simulink model "HLS_VMC_testing"  (R2025a)
settings: Solver=VariableStepAuto  StartTime=0.0  StopTime=0.0001  RelTol=1e-3
InitFcn:
  | fs = 500e6;
values from neighbouring files (symbols this model uses):
  N = length(X)    [outputPlots.m]
undefined symbols (not defined in the file or in its folder): A, es1, i, S, vsva2488, xcvr1602
libraries: hdlBasic x98, hlsBasic x64, aieUtilities x18, dspsrcs4 x15, dspxfrm3 x2, hdlDSPIP x2, hlsUtilities x1, vmcUtilities x1
(part 3 of 4)

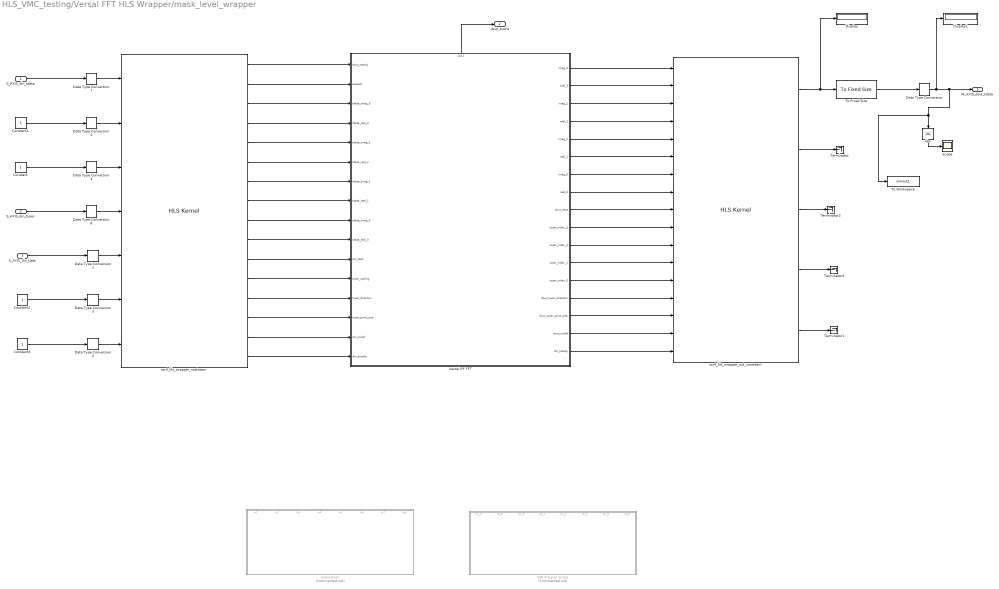
== system HLS_VMC_testing/Versal FFT HLS Wrapper/mask_level_wrapper ==
  S_AXIS_din_tdata : Inport
  S_AXIS_din_tuser : Inport  Port=2
  S_AXIS_din_tlast : Inport  Port=3
  Abs : Abs  SaturateOnIntegerOverflow=off
  Constant{,1..3} (4 alike) : Constant
  Data Type Conversion : hlsBasic/Data Type Conversion  OutDataType=double  TypeExp=''  Signedness=Signed  WordLength=16  FractionalLength=0  RoundingMode=Truncation to minus infinity  OverflowMode=Wrap around
  Data Type Conversion{1..5} (5 alike) : hlsBasic/Data Type Conversion  OutDataType=data type expression  TypeExp='x_ufix1'  Signedness=Signed  WordLength=16  FractionalLength=0  RoundingMode=Truncation to minus infinity  OverflowMode=Wrap around
  Data Type Conversion7 : hlsBasic/Data Type Conversion  OutDataType=data type expression  TypeExp='x_sfix64_En63'  Signedness=Signed  WordLength=16  FractionalLength=0  RoundingMode=Truncation to minus infinity  OverflowMode=Wrap around  SaturateOnIntegerOverflow=on
  Data Type Conversion8 : hlsBasic/Data Type Conversion  OutDataType=data type expression  TypeExp='x_ufix18'  Signedness=Signed  WordLength=16  FractionalLength=0  RoundingMode=Truncation to minus infinity  OverflowMode=Wrap around
  Display : Display
  Display1 : Display
  SSR 4 Signal Scope : Subsystem  Commented=on
  Scope : Scope
      settings: ActiveDisplayYMinimum=-0.036579755749096929  ActiveDisplayYMaximum=0.32921780174187243  DataLoggingVariableName=ScopeData4
  Subsystem : Subsystem  Commented=on
  Terminator{,1..3} (4 alike) : Terminator
  To Fixed Size : aieUtilities/To Fixed Size  Mode=Stop simulation when input variable-size signal is not full  OutputSize=Inherit: Same as input  CopyMethod=Buffer samples to form output  HasStatusOutput=on
  To Workspace : ToWorkspace  VariableName=simout1  SaveFormat=Timeseries  SampleTime=-1
  Versal RF FFT : Subsystem
      settings: PortSchema="{\"entries\":[{\"content\":{\"sides\":[{\"content\":{\"connectorIds\":[\"In1\",\"In2\",\"In3\",\"In4\",\"In5\",\"In6\",\"In7\",\"In8\",\"In9\",\"In10\",\"In11\",\"In12\",\"In13\",\"In14\",\"In15\",\"In16\"]},\"type\":\"ConnectorPlacement.EquallySpacedRectSide\",\"uuid\":\"209a2209-87d3-42b4-b17f-a75cbba28a6a\"},{\"content\":{\"connectorIds\":[\"Out1\",\"Out2\",\"Out3\",\"Out4\",\"Out5\",\"Out6\",\"Out7\",\"Out8\",\"Out9\",\"Out10\",\"Out11\",\"Out12\",\"Out13\",\"Out14\",\"Out15\",\"Out16\",\"Out17\"],\"side\":\"RIGHT\"},\"type\":\"ConnectorPlacement.EquallySpacedRectSide\",\"uuid\":\"ba4fa1b1-993b-4b6c-82ac-7a0960139a7d\"},{\"content\":{\"connectorIds\":[\"Out18\"],\"side\":\"TOP\"},\"type\":\"ConnectorPlacement.EquallySpacedRectSide\",\"uuid\":\"00677fce-2a91-4297-b798-cc966ff20102\"}]},\"type\":\"ConnectorPlacement.EquallySpacedConnector\",\"uuid\":\"b06fffb5-4716-4994-a196-524358a0c89f\"}],\"packageUris\":[\"http://schema.mathworks.com/mf0/Connector/R2020b\"],\"version\":\"1.0\"}"
  ssr4_hls_wrapper_nostream : hlsBasic/HLS Kernel  PortNames={'return'; 'S_AXIS_din_tdata'; 'S_AXIS_din_tready_IN'; 'S_AXIS_din_tvalid_IN'; 'S_AXIS_din_tuser_IN'; 'S_AXIS_din_tlast_IN'; 'S_AXI_aresetn_IN'; 'S_AXI_enable_IN'; 'M_AXIS_dout_tready_OUT'; 'M_AXI_aresetn_OUT'; 'M_AXIS_din_tdata_sample_3_imag'; 'M_AXIS_din_tdata_sample_3_real'; 'M_AXIS_din_tdata_sample_2_imag'; 'M_AXIS_din_tdata_sample_2_real'; 'M_AXIS_din_tdata_sample_1_imag'; 'M_AXIS_din_tdata_sample_1_real'; 'M_AXIS_din_tdata_sample_0_imag'; 'M_AXIS_din_tdata_sample_0_real'; 'M_AXIS_din_tlast_OUT'; 'M_AXIS_din_tuser_scaling'; 'M_AXIS_din_tuser_direction'; 'M_AXIS_din_tuser_point_size'; 'M_AXIS_din_tvalid_OUT'; 'M_AXI_enable_OUT'}  PortSerializedTypes={'{Bv}'; '{R{Tstd::complex{1{t{Tap_fixed{5{t{}64}{t{}1}{t{}5}{t{}3}{t{}0}}}}}}}'; '{R{Tap_uint{1{t{}1}}}}'; '{R{Tap_uint{1{t{}1}}}}'; '{R{Tap_ufixed{5{t{}18}{t{}18}{t{}5}{t{}3}{t{}0}}}}'; '{R{Tap_uint{1{t{}1}}}}'; '{R{Tap_uint{1{t{}1}}}}'; '{R{Tap_uint{1{t{}1}}}}'; '{R{Tap_uint{1{t{}1}}}}'; '{R{Tap_uint{1{t{}1}}}}'; '{R{Tap_fixed{5{t{}16}{t{}1}{t{}0}{t{}3}{t{}0}}}}'; '{R{Tap_fixed{5{t{}16}{t{}1}{t{}0}{t{}3}{t{}0}}}}'; '{R{Tap_fixed{5{t{}16}{t{}1}{t{}0}{t{}3}{t{}0}}}}'; '{R{Tap_fixed{5{t{}16}{t{}1}{t{}0}{t{}3}{t{}0}}}}'; '{R{Tap_fixed{5{t{}16}{t{}1}{t{}0}{t{}3}{t{}0}}}}'; '{R{Tap_fixed{5{t{}16}{t{}1}{t{}0}{t{}3}{t{}0}}}}'; '{R{Tap_fixed{5{t{}16}{t{}1}{t{}0}{t{}3}{t{}0}}}}'; '{R{Tap_fixed{5{t{}16}{t{}1}{t{}0}{t{}3}{t{}0}}}}'; '{R{Tap_uint{1{t{}1}}}}'; '{R{Tap_ufixed{5{t{}13}{t{}1}{t{}5}{t{}3}{t{}0}}}}'; '{R{Tap_uint{1{t{}1}}}}'; '{R{Tap_uint{1{t{}4}}}}'; '{R{Tap_uint{1{t{}1}}}}'; '{R{Tap_uint{1{t{}1}}}}'}  FunctionTemplateSpecKind=none  FunctionTemplateParamNames={}  FunctionTemplateParamKinds={}  FunctionTemplateParamTypes={}  FunctionTemplateParamValues={}  PortSynchronicities={'sync'; 'sync'; 'sync'; 'sync'; 'sync'; 'sync'; 'sync'; 'sync'; 'sync'; 'sync'; 'sync'; 'sync'; 'sync'; 'sync'; 'sync'; 'sync'; 'sync'; 'sync'; 'sync'; 'sync'; 'sync'; 'sync'; 'sync'}  PortSignalSizes={0.000000000000000000e+00; 0.000000000000000000e+00; 0.000000000000000000e+00; 0.000000000000000000e+00; 0.000000000000000000e+00; 0.000000000000000000e+00; 0.000000000000000000e+00; 0.000000000000000000e+00; 0.000000000000000000e+00; 0.000000000000000000e+00; 0.000000000000000000e+00; 0.000000000000000000e+00; 0.000000000000000000e+00; 0.000000000000000000e+00; 0.000000000000000000e+00; 0.000000000000000000e+00; 0.000000000000000000e+00; 0.000000000000000000e+00; 0.000000000000000000e+00; 0.000000000000000000e+00; 0.000000000000000000e+00; 0.000000000000000000e+00; 0.000000000000000000e+00}  PortParameterValues={}  PortAttributesTable={ 'Input', 'S_AXIS_din_tdata', 'std::complex< ap_fixed< 64, 1, 5, 3, 0 > > &', 'sync', ''; 'Input', 'S_AXIS_din_tready_IN', 'ap_uint< 1 > &', 'sync', ''; 'Input', 'S_AXIS_din_tvalid_IN', 'ap_uint< 1 > &', 'sync', ''; 'Input', 'S_AXIS_din_tuser_IN', 'ap_ufixed< 18, 18, 5, 3, 0 > &', 'sync', ''; 'Input', 'S_AXIS_din_tlast_IN', 'ap_uint< 1 > &', 'sync', ''; 'Input', 'S_AXI_aresetn_IN', 'ap_uint< 1 > &', 'sync', ''; 'Input', 'S_AXI_enable_IN', 'ap_uint< 1 > &', 'sync', ''; 'Inout', 'M_AXIS_dout_tready_OUT', 'ap_uint< 1 > &', 'sync', ''; 'Inout', 'M_AXI_aresetn_OUT', 'ap_uint< 1 > &', 'sync', ''; 'Inout', 'M_AXIS_din_tdata_sample_3_imag', 'ap_fixed< 16, 1, 0, 3, 0 > &', 'sync', ''; 'Inout', 'M_AXIS_din_tdata_sample_3_real', 'ap_fixed< 16, 1, 0, 3, 0 > &', 'sync', ''; 'Inout', 'M_AXIS_din_tdata_sample_2_imag', 'ap_fixed< 16, 1, 0, 3, 0 > &', 'sync', ''; 'Inout', 'M_AXIS_din_tdata_sample_2_real', 'ap_fixed< 16, 1, 0, 3, 0 > &', 'sync', ''; 'Inout', 'M_AXIS_din_tdata_sample_1_imag', 'ap_fixed< 16, 1, 0, 3, 0 > &', 'sync', ''; 'Inout', 'M_AXIS_din_tdata_sample_1_real', 'ap_fixed< 16, 1, 0, 3, 0 > &', 'sync', ''; 'Inout', 'M_AXIS_din_tdata_sample_0_imag', 'ap_fixed< 16, 1, 0, 3, 0 > &', 'sync', ''; 'Inout', 'M_AXIS_din_tdata_sample_0_real', 'ap_fixed< 16, 1, 0, 3, 0 > &', 'sync', ''; 'Inout', 'M_AXIS_din_tlast_OUT', 'ap_uint< 1 > &', 'sync', ''; 'Inout', 'M_AXIS_din_tuser_scaling', 'ap_ufixed< 13, 1, 5, 3, 0 > &', 'sync', ''; 'Inout', 'M_AXIS_din_tuser_direction', 'ap_uint< 1 > &', 'sync', ''; 'Inout', 'M_AXIS_din_tuser_point_size', 'ap_uint< 4 > &', 'sync', ''; 'Inout', 'M_AXIS_din_tvalid_OUT', 'ap_uint< 1 > &', 'sync', ''; 'Inout', 'M_AXI_enable_OUT', 'ap_uint< 1 > &', 'sync', '' }  PortAttributesEnablement={'off', 'off', 'off', 'on', 'off';'off', 'off', 'off', 'on', 'off';'off', 'off', 'off', 'on', 'off';'off', 'off', 'off', 'on', 'off';'off', 'off', 'off', 'on', 'off';'off', 'off', 'off', 'on', 'off';'off', 'off', 'off', 'on', 'off';'off', 'off', 'off', 'on', 'off';'off', 'off', 'off', 'on', 'off';'off', 'off', 'off', 'on', 'off';'off', 'off', 'off', 'on', 'off';'off', 'off', 'off', 'on', 'off';'off', 'off', 'off', 'on', 'off';'off', 'off', 'off', 'on', 'off';'off', 'off', 'off', 'on', 'off';'off', 'off', 'off', 'on', 'off';'off', 'off', 'off', 'on', 'off';'off', 'off', 'off', 'on', 'off';'off', 'off', 'off', 'on', 'off';'off', 'off', 'off', 'on', 'off';'off', 'off', 'off', 'on', 'off';'off', 'off', 'off', 'on', 'off';'off', 'off', 'off', 'on', 'off'}  PortParametersTable={}  SampleTime=-1  PortDirectionTable={ 'S_AXIS_din_tdata', 'std::complex< ap_fixed< 64, 1, 5, 3, 0 > > &', 'Input', 'Port'; 'S_AXIS_din_tready_IN', 'ap_uint< 1 > &', 'Input', 'Port'; 'S_AXIS_din_tvalid_IN', 'ap_uint< 1 > &', 'Input', 'Port'; 'S_AXIS_din_tuser_IN', 'ap_ufixed< 18, 18, 5, 3, 0 > &', 'Input', 'Port'; 'S_AXIS_din_tlast_IN', 'ap_uint< 1 > &', 'Input', 'Port'; 'S_AXI_aresetn_IN', 'ap_uint< 1 > &', 'Input', 'Port'; 'S_AXI_enable_IN', 'ap_uint< 1 > &', 'Input', 'Port'; 'M_AXIS_dout_tready_OUT', 'ap_uint< 1 > &', 'Output', 'Port'; 'M_AXI_aresetn_OUT', 'ap_uint< 1 > &', 'Output', 'Port'; 'M_AXIS_din_tdata_sample_3_imag', 'ap_fixed< 16, 1, 0, 3, 0 > &', 'Output', 'Port'; 'M_AXIS_din_tdata_sample_3_real', 'ap_fixed< 16, 1, 0, 3, 0 > &', 'Output', 'Port'; 'M_AXIS_din_tdata_sample_2_imag', 'ap_fixed< 16, 1, 0, 3, 0 > &', 'Output', 'Port'; 'M_AXIS_din_tdata_sample_2_real', 'ap_fixed< 16, 1, 0, 3, 0 > &', 'Output', 'Port'; 'M_AXIS_din_tdata_sample_1_imag', 'ap_fixed< 16, 1, 0, 3, 0 > &', 'Output', 'Port'; 'M_AXIS_din_tdata_sample_1_real', 'ap_fixed< 16, 1, 0, 3, 0 > &', 'Output', 'Port'; 'M_AXIS_din_tdata_sample_0_imag', 'ap_fixed< 16, 1, 0, 3, 0 > &', 'Output', 'Port'; 'M_AXIS_din_tdata_sample_0_real', 'ap_fixed< 16, 1, 0, 3, 0 > &', 'Output', 'Port'; 'M_AXIS_din_tlast_OUT', 'ap_uint< 1 > &', 'Output', 'Port'; 'M_AXIS_din_tuser_scaling', 'ap_ufixed< 13, 1, 5, 3, 0 > &', 'Output', 'Port'; 'M_AXIS_din_tuser_direction', 'ap_uint< 1 > &', 'Output', 'Port'; 'M_AXIS_din_tuser_point_size', 'ap_uint< 4 > &', 'Output', 'Port'; 'M_AXIS_din_tvalid_OUT', 'ap_uint< 1 > &', 'Output', 'Port'; 'M_AXI_enable_OUT', 'ap_uint< 1 > &', 'Output', 'Port' }  FunctionTemplateParams={}  FunctionTemplateParamsEnables={}  FunctionTemplateParamsVisible=off  FunctionDeclTypeOptions=C[1 1]@t7@<empty>  PortDirectionTabVisible=on  ArgDirections={1.000000000000000000e+00; 1.000000000000000000e+00; 1.000000000000000000e+00; 1.000000000000000000e+00; 1.000000000000000000e+00; 1.000000000000000000e+00; 1.000000000000000000e+00; 2.000000000000000000e+00; 2.000000000000000000e+00; 2.000000000000000000e+00; 2.000000000000000000e+00; 2.000000000000000000e+00; 2.000000000000000000e+00; 2.000000000000000000e+00; 2.000000000000000000e+00; 2.000000000000000000e+00; 2.000000000000000000e+00; 2.000000000000000000e+00; 2.000000000000000000e+00; 2.000000000000000000e+00; 2.000000000000000000e+00; 2.000000000000000000e+00; 2.000000000000000000e+00}  ArgInterfaceTypes={1.000000000000000000e+00; 1.000000000000000000e+00; 1.000000000000000000e+00; 1.000000000000000000e+00; 1.000000000000000000e+00; 1.000000000000000000e+00; 1.000000000000000000e+00; 1.000000000000000000e+00; 1.000000000000000000e+00; 1.000000000000000000e+00; 1.000000000000000000e+00; 1.000000000000000000e+00; 1.000000000000000000e+00; 1.000000000000000000e+00; 1.000000000000000000e+00; 1.000000000000000000e+00; 1.000000000000000000e+00; 1.000000000000000000e+00; 1.000000000000000000e+00; 1.000000000000000000e+00; 1.000000000000000000e+00; 1.000000000000000000e+00; 1.000000000000000000e+00}  FunctionIndex=1  FormalArgDecls={'std::complex< ap_fixed< 64, 1, 5, 3, 0 > > & S_AXIS_din_tdata', 'ap_uint< 1 > & S_AXIS_din_tready_IN', 'ap_uint< 1 > & S_AXIS_din_tvalid_IN', 'ap_ufixed< 18, 18, 5, 3, 0 > & S_AXIS_din_tuser_IN', 'ap_uint< 1 > & S_AXIS_din_tlast_IN', 'ap_uint< 1 > & S_AXI_aresetn_IN', 'ap_uint< 1 > & S_AXI_enable_IN', 'ap_uint< 1 > & M_AXIS_dout_tready_OUT', 'ap_uint< 1 > & M_AXI_aresetn_OUT', 'ap_fixed< 16, 1, 0, 3, 0 > & M_AXIS_din_tdata_sample_3_imag', 'ap_fixed< 16, 1, 0, 3, 0 > & M_AXIS_din_tdata_sample_3_real', 'ap_fixed< 16, 1, 0, 3, 0 > & M_AXIS_din_tdata_sample_2_imag', 'ap_fixed< 16, 1, 0, 3, 0 > & M_AXIS_din_tdata_sample_2_real', 'ap_fixed< 16, 1, 0, 3, 0 > & M_AXIS_din_tdata_sample_1_imag', 'ap_fixed< 16, 1, 0, 3, 0 > & M_AXIS_din_tdata_sample_1_real', 'ap_fixed< 16, 1, 0, 3, 0 > & M_AXIS_din_tdata_sample_0_imag', 'ap_fixed< 16, 1, 0, 3, 0 > & M_AXIS_din_tdata_sample_0_real', 'ap_uint< 1 > & M_AXIS_din_tlast_OUT', 'ap_ufixed< 13, 1, 5, 3, 0 > & M_AXIS_din_tuser_scaling', 'ap_uint< 1 > & M_AXIS_din_tuser_direction', 'ap_uint< 4 > & M_AXIS_din_tuser_point_size', 'ap_uint< 1 > & M_AXIS_din_tvalid_OUT', 'ap_uint< 1 > & M_AXI_enable_OUT'}  SimLibPath=''  FunctionTabVisible=on  FunctionDescription=void ssr4_hls_wrapper_nostream(std::complex< ap_fixed< 64, 1, 5, 3, 0 > > & S_AXIS_din_tdata, ap_uint< 1 > & S_AXIS_din_tready_IN, ap_uint< 1 > & S_AXIS_din_tvalid_IN, ap_ufixed< 18, 18, 5, 3, 0 > & S_AXIS_din_tuser_IN, ap_uint< 1 > & S_AXIS_din_tlast_IN, ap_uint< 1 > & S_AXI_aresetn_IN, ap_uint< 1 > & S_AXI_enable_IN, ap_uint< 1 > & M_AXIS_dout_tready_OUT, ap_uint< 1 > & M_AXI_aresetn_OUT, ap_fixed< 16, 1, 0, 3, 0 > & M_AXIS_din_tdata_sample_3_imag, ap_fixed< 16, 1, 0, 3, 0 > & M_AXIS_din_tdata_sample_3_real, ap_fixed< 16, 1, 0, 3, 0 > & M_AXIS_din_tdata_sample_2_imag, ap_fixed< 16, 1, 0, 3, 0 > & M_AXIS_din_tdata_sample_2_real, ap_fixed< 16, 1, 0, 3, 0 > & M_AXIS_din_tdata_sample_1_imag, ap_fixed< 16, 1, 0, 3, 0 > & M_AXIS_din_tdata_sample_1_real, ap_fixed< 16, 1, 0, 3, 0 > & M_AXIS_din_tdata_sample_0_imag, ap_fixed< 16, 1, 0, 3, 0 > & M_AXIS_din_tdata_sample_0_real, ap_uint< 1 > & M_AXIS_din_tlast_OUT, ap_ufixed< 13, 1, 5, 3, 0 > & M_AXIS_din_tuser_scaling, ap_uint< 1 > & M_AXIS_din_tuser_direction, ap_uint< 4 > & M_AXIS_din_tuser_point_size, ap_uint< 1 > & M_AXIS_din_tvalid_OUT, ap_uint< 1 > & M_AXI_enable_OUT)  blockJsonConstraints=[]  deprecateConstraints=0  KernelHeaderFile=src/wrapperin.h  KernelFunction=ssr4_hls_wrapper_nostream  KernelFunctionSelect=<empty>  KernelSourceFile=src/wrapperin.cpp  KernelSearchPaths={}  PreProcOptions={}
  ssr4_hls_wrapper_out_nostream : hlsBasic/HLS Kernel  PortNames={'return'; 'S_AXIS_din_tdata_sample_3_imag'; 'S_AXIS_din_tdata_sample_3_real'; 'S_AXIS_din_tdata_sample_2_imag'; 'S_AXIS_din_tdata_sample_2_real'; 'S_AXIS_din_tdata_sample_1_imag'; 'S_AXIS_din_tdata_sample_1_real'; 'S_AXIS_din_tdata_sample_0_imag'; 'S_AXIS_din_tdata_sample_0_real'; 'S_AXIS_din_tlast_IN'; 'S_AXIS_din_tuser_index_3'; 'S_AXIS_din_tuser_index_2'; 'S_AXIS_din_tuser_index_1'; 'S_AXIS_din_tuser_index_0'; 'S_AXIS_din_tuser_direction'; 'S_AXIS_din_tuser_point_size'; 'S_AXIS_tvalid_IN'; 'S_AXIS_dout_tready_OUT'; 'M_AXIS_dout_tdata'; 'M_AXIS_dout_tlast_OUT'; 'M_AXIS_dout_tready_OUT'; 'M_AXIS_dout_tuser_OUT'; 'M_AXIS_dout_tvalid_OUT'}  PortSerializedTypes={'{Bv}'; '{R{Tap_fixed{5{t{}16}{t{}1}{t{}0}{t{}3}{t{}0}}}}'; '{R{Tap_fixed{5{t{}16}{t{}1}{t{}0}{t{}3}{t{}0}}}}'; '{R{Tap_fixed{5{t{}16}{t{}1}{t{}0}{t{}3}{t{}0}}}}'; '{R{Tap_fixed{5{t{}16}{t{}1}{t{}0}{t{}3}{t{}0}}}}'; '{R{Tap_fixed{5{t{}16}{t{}1}{t{}0}{t{}3}{t{}0}}}}'; '{R{Tap_fixed{5{t{}16}{t{}1}{t{}0}{t{}3}{t{}0}}}}'; '{R{Tap_fixed{5{t{}16}{t{}1}{t{}0}{t{}3}{t{}0}}}}'; '{R{Tap_fixed{5{t{}16}{t{}1}{t{}0}{t{}3}{t{}0}}}}'; '{R{Tap_uint{1{t{}1}}}}'; '{R{Tap_uint{1{t{}12}}}}'; '{R{Tap_uint{1{t{}12}}}}'; '{R{Tap_uint{1{t{}12}}}}'; '{R{Tap_uint{1{t{}12}}}}'; '{R{Tap_uint{1{t{}1}}}}'; '{R{Tap_uint{1{t{}4}}}}'; '{R{Tap_uint{1{t{}1}}}}'; '{R{Tap_uint{1{t{}1}}}}'; '{R{Tstd::complex{1{t{Tap_fixed{5{t{}64}{t{}1}{t{}0}{t{}3}{t{}0}}}}}}}'; '{R{Tap_uint{1{t{}1}}}}'; '{R{Tap_uint{1{t{}1}}}}'; '{R{Tap_uint{1{t{}53}}}}'; '{R{Tap_uint{1{t{}1}}}}'}  FunctionTemplateSpecKind=none  FunctionTemplateParamNames={}  FunctionTemplateParamKinds={}  FunctionTemplateParamTypes={}  FunctionTemplateParamValues={}  PortSynchronicities={'sync'; 'sync'; 'sync'; 'sync'; 'sync'; 'sync'; 'sync'; 'sync'; 'sync'; 'sync'; 'sync'; 'sync'; 'sync'; 'sync'; 'sync'; 'sync'; 'sync'; 'sync'; 'sync'; 'sync'; 'sync'; 'sync'}  PortSignalSizes={0.000000000000000000e+00; 0.000000000000000000e+00; 0.000000000000000000e+00; 0.000000000000000000e+00; 0.000000000000000000e+00; 0.000000000000000000e+00; 0.000000000000000000e+00; 0.000000000000000000e+00; 0.000000000000000000e+00; 0.000000000000000000e+00; 0.000000000000000000e+00; 0.000000000000000000e+00; 0.000000000000000000e+00; 0.000000000000000000e+00; 0.000000000000000000e+00; 0.000000000000000000e+00; 0.000000000000000000e+00; 0.000000000000000000e+00; 0.000000000000000000e+00; 0.000000000000000000e+00; 0.000000000000000000e+00; 0.000000000000000000e+00}  PortParameterValues={}  PortAttributesTable={ 'Input', 'S_AXIS_din_tdata_sample_3_imag', 'ap_fixed< 16, 1, 0, 3, 0 > &', 'sync', ''; 'Input', 'S_AXIS_din_tdata_sample_3_real', 'ap_fixed< 16, 1, 0, 3, 0 > &', 'sync', ''; 'Input', 'S_AXIS_din_tdata_sample_2_imag', 'ap_fixed< 16, 1, 0, 3, 0 > &', 'sync', ''; 'Input', 'S_AXIS_din_tdata_sample_2_real', 'ap_fixed< 16, 1, 0, 3, 0 > &', 'sync', ''; 'Input', 'S_AXIS_din_tdata_sample_1_imag', 'ap_fixed< 16, 1, 0, 3, 0 > &', 'sync', ''; 'Input', 'S_AXIS_din_tdata_sample_1_real', 'ap_fixed< 16, 1, 0, 3, 0 > &', 'sync', ''; 'Input', 'S_AXIS_din_tdata_sample_0_imag', 'ap_fixed< 16, 1, 0, 3, 0 > &', 'sync', ''; 'Input', 'S_AXIS_din_tdata_sample_0_real', 'ap_fixed< 16, 1, 0, 3, 0 > &', 'sync', ''; 'Input', 'S_AXIS_din_tlast_IN', 'ap_uint< 1 > &', 'sync', ''; 'Input', 'S_AXIS_din_tuser_index_3', 'ap_uint< 12 > &', 'sync', ''; 'Input', 'S_AXIS_din_tuser_index_2', 'ap_uint< 12 > &', 'sync', ''; 'Input', 'S_AXIS_din_tuser_index_1', 'ap_uint< 12 > &', 'sync', ''; 'Input', 'S_AXIS_din_tuser_index_0', 'ap_uint< 12 > &', 'sync', ''; 'Input', 'S_AXIS_din_tuser_direction', 'ap_uint< 1 > &', 'sync', ''; 'Input', 'S_AXIS_din_tuser_point_size', 'ap_uint< 4 > &', 'sync', ''; 'Input', 'S_AXIS_tvalid_IN', 'ap_uint< 1 > &', 'sync', ''; 'Input', 'S_AXIS_dout_tready_OUT', 'ap_uint< 1 > &', 'sync', ''; 'Inout', 'M_AXIS_dout_tdata', 'std::complex< ap_fixed< 64, 1, 0, 3, 0 > > &', 'sync', ''; 'Inout', 'M_AXIS_dout_tlast_OUT', 'ap_uint< 1 > &', 'sync', ''; 'Inout', 'M_AXIS_dout_tready_OUT', 'ap_uint< 1 > &', 'sync', ''; 'Inout', 'M_AXIS_dout_tuser_OUT', 'ap_uint< 53 > &', 'sync', ''; 'Inout', 'M_AXIS_dout_tvalid_OUT', 'ap_uint< 1 > &', 'sync', '' }  PortAttributesEnablement={'off', 'off', 'off', 'on', 'off';'off', 'off', 'off', 'on', 'off';'off', 'off', 'off', 'on', 'off';'off', 'off', 'off', 'on', 'off';'off', 'off', 'off', 'on', 'off';'off', 'off', 'off', 'on', 'off';'off', 'off', 'off', 'on', 'off';'off', 'off', 'off', 'on', 'off';'off', 'off', 'off', 'on', 'off';'off', 'off', 'off', 'on', 'off';'off', 'off', 'off', 'on', 'off';'off', 'off', 'off', 'on', 'off';'off', 'off', 'off', 'on', 'off';'off', 'off', 'off', 'on', 'off';'off', 'off', 'off', 'on', 'off';'off', 'off', 'off', 'on', 'off';'off', 'off', 'off', 'on', 'off';'off', 'off', 'off', 'on', 'off';'off', 'off', 'off', 'on', 'off';'off', 'off', 'off', 'on', 'off';'off', 'off', 'off', 'on', 'off';'off', 'off', 'off', 'on', 'off'}  PortParametersTable={}  SampleTime=-1  PortDirectionTable={ 'S_AXIS_din_tdata_sample_3_imag', 'ap_fixed< 16, 1, 0, 3, 0 > &', 'Input', 'Port'; 'S_AXIS_din_tdata_sample_3_real', 'ap_fixed< 16, 1, 0, 3, 0 > &', 'Input', 'Port'; 'S_AXIS_din_tdata_sample_2_imag', 'ap_fixed< 16, 1, 0, 3, 0 > &', 'Input', 'Port'; 'S_AXIS_din_tdata_sample_2_real', 'ap_fixed< 16, 1, 0, 3, 0 > &', 'Input', 'Port'; 'S_AXIS_din_tdata_sample_1_imag', 'ap_fixed< 16, 1, 0, 3, 0 > &', 'Input', 'Port'; 'S_AXIS_din_tdata_sample_1_real', 'ap_fixed< 16, 1, 0, 3, 0 > &', 'Input', 'Port'; 'S_AXIS_din_tdata_sample_0_imag', 'ap_fixed< 16, 1, 0, 3, 0 > &', 'Input', 'Port'; 'S_AXIS_din_tdata_sample_0_real', 'ap_fixed< 16, 1, 0, 3, 0 > &', 'Input', 'Port'; 'S_AXIS_din_tlast_IN', 'ap_uint< 1 > &', 'Input', 'Port'; 'S_AXIS_din_tuser_index_3', 'ap_uint< 12 > &', 'Input', 'Port'; 'S_AXIS_din_tuser_index_2', 'ap_uint< 12 > &', 'Input', 'Port'; 'S_AXIS_din_tuser_index_1', 'ap_uint< 12 > &', 'Input', 'Port'; 'S_AXIS_din_tuser_index_0', 'ap_uint< 12 > &', 'Input', 'Port'; 'S_AXIS_din_tuser_direction', 'ap_uint< 1 > &', 'Input', 'Port'; 'S_AXIS_din_tuser_point_size', 'ap_uint< 4 > &', 'Input', 'Port'; 'S_AXIS_tvalid_IN', 'ap_uint< 1 > &', 'Input', 'Port'; 'S_AXIS_dout_tready_OUT', 'ap_uint< 1 > &', 'Input', 'Port'; 'M_AXIS_dout_tdata', 'std::complex< ap_fixed< 64, 1, 0, 3, 0 > > &', 'Output', 'Port'; 'M_AXIS_dout_tlast_OUT', 'ap_uint< 1 > &', 'Output', 'Port'; 'M_AXIS_dout_tready_OUT', 'ap_uint< 1 > &', 'Output', 'Port'; 'M_AXIS_dout_tuser_OUT', 'ap_uint< 53 > &', 'Output', 'Port'; 'M_AXIS_dout_tvalid_OUT', 'ap_uint< 1 > &', 'Output', 'Port' }  FunctionTemplateParams={}  FunctionTemplateParamsEnables={}  FunctionTemplateParamsVisible=off  FunctionDeclTypeOptions=C[1 1]@t7@<empty>  PortDirectionTabVisible=on  ArgDirections={1.000000000000000000e+00; 1.000000000000000000e+00; 1.000000000000000000e+00; 1.000000000000000000e+00; 1.000000000000000000e+00; 1.000000000000000000e+00; 1.000000000000000000e+00; 1.000000000000000000e+00; 1.000000000000000000e+00; 1.000000000000000000e+00; 1.000000000000000000e+00; 1.000000000000000000e+00; 1.000000000000000000e+00; 1.000000000000000000e+00; 1.000000000000000000e+00; 1.000000000000000000e+00; 1.000000000000000000e+00; 2.000000000000000000e+00; 2.000000000000000000e+00; 2.000000000000000000e+00; 2.000000000000000000e+00; 2.000000000000000000e+00}  ArgInterfaceTypes={1.000000000000000000e+00; 1.000000000000000000e+00; 1.000000000000000000e+00; 1.000000000000000000e+00; 1.000000000000000000e+00; 1.000000000000000000e+00; 1.000000000000000000e+00; 1.000000000000000000e+00; 1.000000000000000000e+00; 1.000000000000000000e+00; 1.000000000000000000e+00; 1.000000000000000000e+00; 1.000000000000000000e+00; 1.000000000000000000e+00; 1.000000000000000000e+00; 1.000000000000000000e+00; 1.000000000000000000e+00; 1.000000000000000000e+00; 1.000000000000000000e+00; 1.000000000000000000e+00; 1.000000000000000000e+00; 1.000000000000000000e+00}  FunctionIndex=1  FormalArgDecls={'ap_fixed< 16, 1, 0, 3, 0 > & S_AXIS_din_tdata_sample_3_imag', 'ap_fixed< 16, 1, 0, 3, 0 > & S_AXIS_din_tdata_sample_3_real', 'ap_fixed< 16, 1, 0, 3, 0 > & S_AXIS_din_tdata_sample_2_imag', 'ap_fixed< 16, 1, 0, 3, 0 > & S_AXIS_din_tdata_sample_2_real', 'ap_fixed< 16, 1, 0, 3, 0 > & S_AXIS_din_tdata_sample_1_imag', 'ap_fixed< 16, 1, 0, 3, 0 > & S_AXIS_din_tdata_sample_1_real', 'ap_fixed< 16, 1, 0, 3, 0 > & S_AXIS_din_tdata_sample_0_imag', 'ap_fixed< 16, 1, 0, 3, 0 > & S_AXIS_din_tdata_sample_0_real', 'ap_uint< 1 > & S_AXIS_din_tlast_IN', 'ap_uint< 12 > & S_AXIS_din_tuser_index_3', 'ap_uint< 12 > & S_AXIS_din_tuser_index_2', 'ap_uint< 12 > & S_AXIS_din_tuser_index_1', 'ap_uint< 12 > & S_AXIS_din_tuser_index_0', 'ap_uint< 1 > & S_AXIS_din_tuser_direction', 'ap_uint< 4 > & S_AXIS_din_tuser_point_size', 'ap_uint< 1 > & S_AXIS_tvalid_IN', 'ap_uint< 1 > & S_AXIS_dout_tready_OUT', 'std::complex< ap_fixed< 64, 1, 0, 3, 0 > > & M_AXIS_dout_tdata', 'ap_uint< 1 > & M_AXIS_dout_tlast_OUT', 'ap_uint< 1 > & M_AXIS_dout_tready_OUT', 'ap_uint< 53 > & M_AXIS_dout_tuser_OUT', 'ap_uint< 1 > & M_AXIS_dout_tvalid_OUT'}  SimLibPath=''  FunctionTabVisible=on  FunctionDescription=void ssr4_hls_wrapper_out_nostream(ap_fixed< 16, 1, 0, 3, 0 > & S_AXIS_din_tdata_sample_3_imag, ap_fixed< 16, 1, 0, 3, 0 > & S_AXIS_din_tdata_sample_3_real, ap_fixed< 16, 1, 0, 3, 0 > & S_AXIS_din_tdata_sample_2_imag, ap_fixed< 16, 1, 0, 3, 0 > & S_AXIS_din_tdata_sample_2_real, ap_fixed< 16, 1, 0, 3, 0 > & S_AXIS_din_tdata_sample_1_imag, ap_fixed< 16, 1, 0, 3, 0 > & S_AXIS_din_tdata_sample_1_real, ap_fixed< 16, 1, 0, 3, 0 > & S_AXIS_din_tdata_sample_0_imag, ap_fixed< 16, 1, 0, 3, 0 > & S_AXIS_din_tdata_sample_0_real, ap_uint< 1 > & S_AXIS_din_tlast_IN, ap_uint< 12 > & S_AXIS_din_tuser_index_3, ap_uint< 12 > & S_AXIS_din_tuser_index_2, ap_uint< 12 > & S_AXIS_din_tuser_index_1, ap_uint< 12 > & S_AXIS_din_tuser_index_0, ap_uint< 1 > & S_AXIS_din_tuser_direction, ap_uint< 4 > & S_AXIS_din_tuser_point_size, ap_uint< 1 > & S_AXIS_tvalid_IN, ap_uint< 1 > & S_AXIS_dout_tready_OUT, std::complex< ap_fixed< 64, 1, 0, 3, 0 > > & M_AXIS_dout_tdata, ap_uint< 1 > & M_AXIS_dout_tlast_OUT, ap_uint< 1 > & M_AXIS_dout_tready_OUT, ap_uint< 53 > & M_AXIS_dout_tuser_OUT, ap_uint< 1 > & M_AXIS_dout_tvalid_OUT)  blockJsonConstraints=[]  deprecateConstraints=0  KernelHeaderFile=wrapper_out_src/wrapperout.h  KernelFunction=ssr4_hls_wrapper_out_nostream  KernelFunctionSelect=<empty>  KernelSourceFile=wrapper_out_src/wrapperout.cpp  KernelSearchPaths={}  PreProcOptions={}
  M_AXIS_dout_tdata : Outport
  dout_tvalid : Outport  Port=2
  wires:
  Versal RF FFT/17(din_tready) -> ssr4_hls_wrapper_out_nostream/17
  ssr4_hls_wrapper_out_nostream/1 -> Display/1, To Fixed Size/1
  Data Type Conversion7/1 -> ssr4_hls_wrapper_nostream/1
  To Fixed Size/1 -> Data Type Conversion/1
  Versal RF FFT/16(dout_tvalid) -> ssr4_hls_wrapper_out_nostream/16
  Versal RF FFT/15(dout_tuser_point_size) -> ssr4_hls_wrapper_out_nostream/15
  Versal RF FFT/14(dout_tuser_direction) -> ssr4_hls_wrapper_out_nostream/14
  Versal RF FFT/13(tuser_index_0) -> ssr4_hls_wrapper_out_nostream/13
  Versal RF FFT/9(dout_tlast) -> ssr4_hls_wrapper_out_nostream/9
  Versal RF FFT/8(real_0) -> ssr4_hls_wrapper_out_nostream/8
  Versal RF FFT/7(imag_0) -> ssr4_hls_wrapper_out_nostream/7
  Versal RF FFT/6(real_1) -> ssr4_hls_wrapper_out_nostream/6
  Versal RF FFT/5(imag_1) -> ssr4_hls_wrapper_out_nostream/5
  Versal RF FFT/4(real_2) -> ssr4_hls_wrapper_out_nostream/4
  Versal RF FFT/3(imag_2) -> ssr4_hls_wrapper_out_nostream/3
  Versal RF FFT/1(imag_3) -> ssr4_hls_wrapper_out_nostream/1
  Versal RF FFT/2(real_3) -> ssr4_hls_wrapper_out_nostream/2
  Versal RF FFT/10(tuser_index_3) -> ssr4_hls_wrapper_out_nostream/10
  Versal RF FFT/11(tuser_index_2) -> ssr4_hls_wrapper_out_nostream/11
  Versal RF FFT/12(tuser_index_1) -> ssr4_hls_wrapper_out_nostream/12
  S_AXIS_din_tdata/1 -> Data Type Conversion7/1
  ssr4_hls_wrapper_nostream/1 -> Versal RF FFT/1(dout_tready)
  ssr4_hls_wrapper_nostream/2 -> Versal RF FFT/2(aresetn)
  ssr4_hls_wrapper_nostream/3 -> Versal RF FFT/3(tdata_imag_3)
  ssr4_hls_wrapper_nostream/4 -> Versal RF FFT/4(tdata_real_3)
  ssr4_hls_wrapper_nostream/5 -> Versal RF FFT/5(tdata_imag_2)
  ssr4_hls_wrapper_nostream/6 -> Versal RF FFT/6(tdata_real_2)
  ssr4_hls_wrapper_nostream/7 -> Versal RF FFT/7(tdata_imag_1)
  ssr4_hls_wrapper_nostream/8 -> Versal RF FFT/8(tdata_real_1)
  ssr4_hls_wrapper_nostream/9 -> Versal RF FFT/9(tdata_imag_0)
  ssr4_hls_wrapper_nostream/10 -> Versal RF FFT/10(tdata_real_0)
  ssr4_hls_wrapper_nostream/11 -> Versal RF FFT/11(din_tlast)
  ssr4_hls_wrapper_nostream/12 -> Versal RF FFT/12(tuser_scaling)
  ssr4_hls_wrapper_nostream/13 -> Versal RF FFT/13(tuser_direction)
  ssr4_hls_wrapper_nostream/14 -> Versal RF FFT/14(tuser_point_size)
  ssr4_hls_wrapper_nostream/15 -> Versal RF FFT/15(din_tvalid)
  ssr4_hls_wrapper_nostream/16 -> Versal RF FFT/16(din_enable)
  Versal RF FFT/18(Out1) -> dout_tvalid/1
  Data Type Conversion/1 -> Display1/1, To Workspace/1, Abs/1, M_AXIS_dout_tdata/1
  Abs/1 -> Scope/1
  ssr4_hls_wrapper_out_nostream/2 -> Terminator/1
  ssr4_hls_wrapper_out_nostream/4 -> Terminator3/1
  ssr4_hls_wrapper_out_nostream/3 -> Terminator2/1
  ssr4_hls_wrapper_out_nostream/5 -> Terminator1/1
  Data Type Conversion8/1 -> ssr4_hls_wrapper_nostream/4
  S_AXIS_din_tuser/1 -> Data Type Conversion8/1
  Constant/1 -> Data Type Conversion4/1
  Constant2/1 -> Data Type Conversion3/1
  Constant3/1 -> Data Type Conversion2/1
  Data Type Conversion1/1 -> ssr4_hls_wrapper_nostream/5
  S_AXIS_din_tlast/1 -> Data Type Conversion1/1
  Constant1/1 -> Data Type Conversion5/1
  Data Type Conversion2/1 -> ssr4_hls_wrapper_nostream/7
  Data Type Conversion3/1 -> ssr4_hls_wrapper_nostream/6
  Data Type Conversion5/1 -> ssr4_hls_wrapper_nostream/2
  Data Type Conversion4/1 -> ssr4_hls_wrapper_nostream/3

== system HLS_VMC_testing/Versal FFT HLS Wrapper1/TUSER formatting ==
  In1 : Inport
  In2 : Inport  Port=2
  In3 : Inport  Port=3
  Concat : hdlBasic/Concat  num_inputs=3  XmcBlockStatus=1  maskContainerNames=group1  block_type=concat  block_config=sysgen:Concat_config
  Gateway In : hdlBasic/Gateway In  gui_display_data_type=Fixed-point  arith_type=Unsigned  n_bits=13  bin_pt=13  preci_type=Single  exp_width=8  frac_width=24  rows=1  columns=1  quantization="Round  (unbiased: +/- Inf)"  overflow=Saturate  period=1/fs  UseAsADC=off  ADCChannel='1'  interface=None  automatic_assignment=on  address_offset=hex2dec('00')  intf_name=''  intf_description=''  default_value=0  timing_constraint=None  locs_specified=off  LOCs={}  io_standard={}  inherit_from_input=off  hdl_port=on  XmcBlockStatus=1  maskContainerNames=group4  block_type=gatewayin  block_config=sysgen:gateway_in_config  block_width_w=590  block_height_w=620  block_width=640  block_height=850
  Gateway In1 : hdlBasic/Gateway In  gui_display_data_type=Boolean  arith_type=Boolean  n_bits=16  bin_pt=14  preci_type=Single  exp_width=8  frac_width=24  rows=1  columns=1  quantization="Round  (unbiased: +/- Inf)"  overflow=Saturate  period=1/fs  UseAsADC=off  ADCChannel='1'  interface=None  automatic_assignment=on  address_offset=hex2dec('00')  intf_name=''  intf_description=''  default_value=0  timing_constraint=None  locs_specified=off  LOCs={}  io_standard={}  inherit_from_input=off  hdl_port=on  XmcBlockStatus=1  maskContainerNames=group4  block_type=gatewayin  block_config=sysgen:gateway_in_config  block_width_w=590  block_height_w=620  block_width=640  block_height=850
  Gateway In2 : hdlBasic/Gateway In  gui_display_data_type=Fixed-point  arith_type=Unsigned  n_bits=4  bin_pt=0  preci_type=Single  exp_width=8  frac_width=24  rows=1  columns=1  quantization="Round  (unbiased: +/- Inf)"  overflow=Saturate  period=1/fs  UseAsADC=off  ADCChannel='1'  interface=None  automatic_assignment=on  address_offset=hex2dec('00')  intf_name=''  intf_description=''  default_value=0  timing_constraint=None  locs_specified=off  LOCs={}  io_standard={}  inherit_from_input=off  hdl_port=on  XmcBlockStatus=1  maskContainerNames=group4  block_type=gatewayin  block_config=sysgen:gateway_in_config  block_width_w=590  block_height_w=620  block_width=640  block_height=850
  Gateway Out : hdlBasic/Gateway Out  inherit_from_input=off  bool_to_boolean=off  hdl_port=on  rows=1  columns=1  UseAsDAC=off  DACChannel='1'  interface=None  automatic_assignment=on  address_offset=hex2dec('00')  intf_name=''  intf_description=''  timing_constraint=None  locs_specified=off  LOCs={}  io_standard={}  XmcBlockStatus=1  maskContainerNames=group4  block_type=gatewayout  block_config=sysgen:gateway_out_config  block_width_w=590  block_height_w=620  block_width=620  block_height=750
  Shift : hdlBasic/Shift  shift_dir=Left  shift_bits=13  en=off  latency=0  precision=User Defined  arith_type=Unsigned  n_bits=13  bin_pt=0  quantization=Truncate  overflow=Wrap  XmcBlockStatus=1  maskContainerNames=group2  block_type=shift  block_config=sysgen:Shift_config
  S_AXIS_din_tuser_ : Outport
  wires:
  Concat/1 -> Gateway Out/1
  In1/1 -> Gateway In/1
  In2/1 -> Gateway In1/1
  In3/1 -> Gateway In2/1
  Gateway In/1 -> Shift/1
  Gateway In2/1 -> Concat/3
  Gateway In1/1 -> Concat/2
  Gateway Out/1 -> S_AXIS_din_tuser_/1
  Shift/1 -> Concat/1

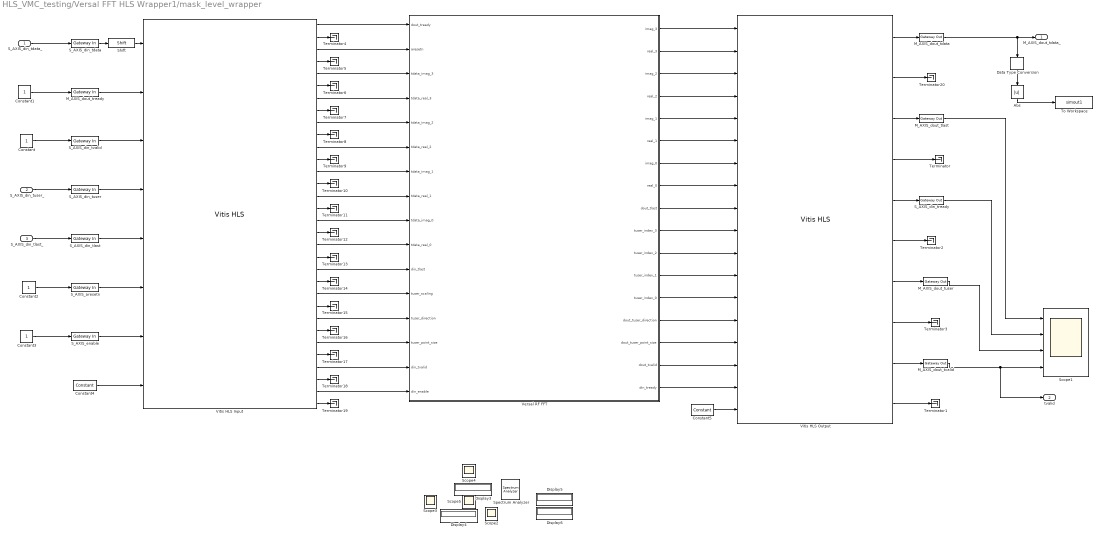
== system HLS_VMC_testing/Versal FFT HLS Wrapper1/mask_level_wrapper ==
  S_AXIS_din_tdata_ : Inport
  S_AXIS_din_tuser_ : Inport  Port=2
  S_AXIS_din_tlast_ : Inport  Port=3
  Abs : Abs  SaturateOnIntegerOverflow=off
  Constant{,1..3} (4 alike) : Constant
  Constant4 : hdlBasic/Constant  const=0  gui_display_data_type=Boolean  arith_type=Boolean  n_bits=16  bin_pt=14  preci_type=Single  exp_width=8  frac_width=24  explicit_period=off  period=1  XmcBlockStatus=1  maskContainerNames=tabcontainer1  block_type=constant  block_config=sysgen:Constant_config
  Constant5 : hdlBasic/Constant  const=0  gui_display_data_type=Boolean  arith_type=Boolean  n_bits=16  bin_pt=14  preci_type=Single  exp_width=8  frac_width=24  explicit_period=off  period=1  XmcBlockStatus=1  maskContainerNames=tabcontainer1  block_type=constant  block_config=sysgen:Constant_config
  Data Type Conversion : hlsBasic/Data Type Conversion  OutDataType=double  TypeExp=''  Signedness=Signed  WordLength=16  FractionalLength=0  RoundingMode=Truncation to minus infinity  OverflowMode=Wrap around
  Display{3..6} (4 alike) : Display
  M_AXIS_dout_tdata : hdlBasic/Gateway Out  inherit_from_input=off  bool_to_boolean=off  hdl_port=on  rows=1  columns=1  UseAsDAC=off  DACChannel='1'  interface=None  automatic_assignment=on  address_offset=hex2dec('00')  intf_name=''  intf_description=''  timing_constraint=None  locs_specified=off  LOCs={}  io_standard={}  XmcBlockStatus=1  maskContainerNames=group4  block_type=gatewayout  block_config=sysgen:gateway_out_config  block_width_w=590  block_height_w=620  block_width=620  block_height=750
  M_AXIS_dout_tlast : hdlBasic/Gateway Out  inherit_from_input=off  bool_to_boolean=off  hdl_port=on  rows=1  columns=1  UseAsDAC=off  DACChannel='1'  interface=None  automatic_assignment=on  address_offset=hex2dec('00')  intf_name=''  intf_description=''  timing_constraint=None  locs_specified=off  LOCs={}  io_standard={}  XmcBlockStatus=1  maskContainerNames=group4  block_type=gatewayout  block_config=sysgen:gateway_out_config  block_width_w=590  block_height_w=620  block_width=620  block_height=750
  M_AXIS_dout_tready : hdlBasic/Gateway In  gui_display_data_type=Boolean  arith_type=Boolean  n_bits=16  bin_pt=14  preci_type=Single  exp_width=8  frac_width=24  rows=1  columns=1  quantization="Round  (unbiased: +/- Inf)"  overflow=Saturate  period=1/fs  UseAsADC=off  ADCChannel='1'  interface=None  automatic_assignment=on  address_offset=hex2dec('00')  intf_name=''  intf_description=''  default_value=0  timing_constraint=None  locs_specified=off  LOCs={}  io_standard={}  inherit_from_input=off  hdl_port=on  XmcBlockStatus=1  maskContainerNames=group4  block_type=gatewayin  block_config=sysgen:gateway_in_config  block_width_w=590  block_height_w=620  block_width=640  block_height=850
  M_AXIS_dout_tuser : hdlBasic/Gateway Out  inherit_from_input=off  bool_to_boolean=off  hdl_port=on  rows=1  columns=1  UseAsDAC=off  DACChannel='1'  interface=None  automatic_assignment=on  address_offset=hex2dec('00')  intf_name=''  intf_description=''  timing_constraint=None  locs_specified=off  LOCs={}  io_standard={}  XmcBlockStatus=1  maskContainerNames=group4  block_type=gatewayout  block_config=sysgen:gateway_out_config  block_width_w=590  block_height_w=620  block_width=620  block_height=750
  M_AXIS_dout_tvalid : hdlBasic/Gateway Out  inherit_from_input=off  bool_to_boolean=off  hdl_port=on  rows=1  columns=1  UseAsDAC=off  DACChannel='1'  interface=None  automatic_assignment=on  address_offset=hex2dec('00')  intf_name=''  intf_description=''  timing_constraint=None  locs_specified=off  LOCs={}  io_standard={}  XmcBlockStatus=1  maskContainerNames=group4  block_type=gatewayout  block_config=sysgen:gateway_out_config  block_width_w=590  block_height_w=620  block_width=620  block_height=750
  S_AXIS_aresetn : hdlBasic/Gateway In  gui_display_data_type=Boolean  arith_type=Boolean  n_bits=16  bin_pt=14  preci_type=Single  exp_width=8  frac_width=24  rows=1  columns=1  quantization="Round  (unbiased: +/- Inf)"  overflow=Saturate  period=1/fs  UseAsADC=off  ADCChannel='1'  interface=None  automatic_assignment=on  address_offset=hex2dec('00')  intf_name=''  intf_description=''  default_value=0  timing_constraint=None  locs_specified=off  LOCs={}  io_standard={}  inherit_from_input=off  hdl_port=on  XmcBlockStatus=1  maskContainerNames=group4  block_type=gatewayin  block_config=sysgen:gateway_in_config  block_width_w=590  block_height_w=620  block_width=640  block_height=850
  S_AXIS_din_tdata : hdlBasic/Gateway In  gui_display_data_type=Fixed-point  arith_type=Signed (2's comp)  n_bits=128  bin_pt=127  preci_type=Single  exp_width=8  frac_width=24  rows=1  columns=1  quantization="Round  (unbiased: +/- Inf)"  overflow=Saturate  period=1/fs  UseAsADC=off  ADCChannel='1'  interface=None  automatic_assignment=on  address_offset=hex2dec('00')  intf_name=''  intf_description=''  default_value=0  timing_constraint=None  locs_specified=off  LOCs={}  io_standard={}  inherit_from_input=off  hdl_port=on  XmcBlockStatus=1  maskContainerNames=group4  block_type=gatewayin  block_config=sysgen:gateway_in_config  block_width_w=590  block_height_w=620  block_width=640  block_height=850
  S_AXIS_din_tlast : hdlBasic/Gateway In  gui_display_data_type=Boolean  arith_type=Boolean  n_bits=16  bin_pt=14  preci_type=Single  exp_width=8  frac_width=24  rows=1  columns=1  quantization="Round  (unbiased: +/- Inf)"  overflow=Saturate  period=1/fs  UseAsADC=off  ADCChannel='1'  interface=None  automatic_assignment=on  address_offset=hex2dec('00')  intf_name=''  intf_description=''  default_value=0  timing_constraint=None  locs_specified=off  LOCs={}  io_standard={}  inherit_from_input=off  hdl_port=on  XmcBlockStatus=1  maskContainerNames=group4  block_type=gatewayin  block_config=sysgen:gateway_in_config  block_width_w=590  block_height_w=620  block_width=640  block_height=850
  S_AXIS_din_tready : hdlBasic/Gateway Out  inherit_from_input=off  bool_to_boolean=off  hdl_port=on  rows=1  columns=1  UseAsDAC=off  DACChannel='1'  interface=None  automatic_assignment=on  address_offset=hex2dec('00')  intf_name=''  intf_description=''  timing_constraint=None  locs_specified=off  LOCs={}  io_standard={}  XmcBlockStatus=1  maskContainerNames=group4  block_type=gatewayout  block_config=sysgen:gateway_out_config  block_width_w=590  block_height_w=620  block_width=620  block_height=750
  S_AXIS_din_tuser : hdlBasic/Gateway In  gui_display_data_type=Fixed-point  arith_type=Unsigned  n_bits=18  bin_pt=0  preci_type=Single  exp_width=8  frac_width=24  rows=1  columns=1  quantization="Round  (unbiased: +/- Inf)"  overflow=Saturate  period=1/fs  UseAsADC=off  ADCChannel='1'  interface=None  automatic_assignment=on  address_offset=hex2dec('00')  intf_name=''  intf_description=''  default_value=0  timing_constraint=None  locs_specified=off  LOCs={}  io_standard={}  inherit_from_input=off  hdl_port=on  XmcBlockStatus=1  maskContainerNames=group4  block_type=gatewayin  block_config=sysgen:gateway_in_config  block_width_w=590  block_height_w=620  block_width=640  block_height=850
  S_AXIS_din_tvalid : hdlBasic/Gateway In  gui_display_data_type=Boolean  arith_type=Boolean  n_bits=16  bin_pt=14  preci_type=Single  exp_width=8  frac_width=24  rows=1  columns=1  quantization="Round  (unbiased: +/- Inf)"  overflow=Saturate  period=1/fs  UseAsADC=off  ADCChannel='1'  interface=None  automatic_assignment=on  address_offset=hex2dec('00')  intf_name=''  intf_description=''  default_value=0  timing_constraint=None  locs_specified=off  LOCs={}  io_standard={}  inherit_from_input=off  hdl_port=on  XmcBlockStatus=1  maskContainerNames=group4  block_type=gatewayin  block_config=sysgen:gateway_in_config  block_width_w=590  block_height_w=620  block_width=640  block_height=850
  S_AXIS_enable : hdlBasic/Gateway In  gui_display_data_type=Boolean  arith_type=Boolean  n_bits=16  bin_pt=14  preci_type=Single  exp_width=8  frac_width=24  rows=1  columns=1  quantization="Round  (unbiased: +/- Inf)"  overflow=Saturate  period=1/fs  UseAsADC=off  ADCChannel='1'  interface=None  automatic_assignment=on  address_offset=hex2dec('00')  intf_name=''  intf_description=''  default_value=0  timing_constraint=None  locs_specified=off  LOCs={}  io_standard={}  inherit_from_input=off  hdl_port=on  XmcBlockStatus=1  maskContainerNames=group4  block_type=gatewayin  block_config=sysgen:gateway_in_config  block_width_w=590  block_height_w=620  block_width=640  block_height=850
  Scope1 : Scope  NumInputPorts=4
      settings: ActiveDisplayYMinimum=-0.12499999999999997  ActiveDisplayYMaximum=1.125  DataLoggingVariableName=ScopeData11
  Scope{2..5} (4 alike) : Scope
      Scope2 settings: ActiveDisplayYMinimum=-1.7612064540296718E+38  ActiveDisplayYMaximum=2.0861472000085103E+38  DataLoggingVariableName=ScopeData14
      Scope3 settings: DataLoggingVariableName=ScopeData19
      Scope4 settings: ActiveDisplayYMinimum=-1  ActiveDisplayYMaximum=1  DataLoggingVariableName=ScopeData20
      Scope5 settings: ActiveDisplayYMinimum=-1  ActiveDisplayYMaximum=1  DataLoggingVariableName=ScopeData21
  Shift : hdlBasic/Shift  shift_dir=Left  shift_bits=127  en=off  latency=0  precision=User Defined  arith_type="Signed  (2's comp)"  n_bits=128  bin_pt=0  quantization="Round  (unbiased: +/- Inf)"  overflow=Saturate  XmcBlockStatus=1  maskContainerNames=group2  block_type=shift  block_config=sysgen:Shift_config
  Spectrum Analyzer : SpectrumAnalyzer  WindowPosition=[546.000000,274.000000,800.000000,500.000000,]  ScopeFrameLocation=window  WindowInvariantSamplesPerUpdate=on  Span=499999999.99999994  StartFrequency=-249999999.99999997  StopFrequency=249999999.99999997  YLimits=[723.7247 779.8592]
  Terminator{,1..20} (21 alike) : Terminator
  To Workspace : ToWorkspace  VariableName=simout1  SaveFormat=Timeseries  SampleTime=-1
  Versal RF FFT : Subsystem
  Vitis HLS Input : hdlBasic/Vitis HLS  anytable='./HLS/new_wrapperIN/wrapperin/wrapperin/hls'  fast_sim=off  display_datatype=on  rate_propagation_method=Simulink system period  model_file_path=''  latency=1  block_type=vitis_hls
      settings: infoedit=This block allows including C,C++ and SystemC source files in System Generator for DSP designs.
  Vitis HLS Output : hdlBasic/Vitis HLS  anytable='./HLS/wrapper_out/wrapper_out/wrapper_out/hls'  fast_sim=off  display_datatype=off  rate_propagation_method=Simulink system period  model_file_path=''  latency=1  block_type=vitis_hls
      settings: infoedit=This block allows including C,C++ and SystemC source files in System Generator for DSP designs.
  M_AXIS_dout_tdata_ : Outport
  tvalid : Outport  Port=2
  wires:
  Vitis HLS Output/1 -> M_AXIS_dout_tdata/1
  S_AXIS_din_tdata_/1 -> S_AXIS_din_tdata/1
  M_AXIS_dout_tdata/1 -> Data Type Conversion/1, M_AXIS_dout_tdata_/1
  Abs/1 -> To Workspace/1
  Vitis HLS Output/4 -> Terminator/1
  Vitis HLS Output/8 -> Terminator3/1
  Vitis HLS Output/6 -> Terminator2/1
  Vitis HLS Output/10 -> Terminator1/1
  S_AXIS_din_tuser_/1 -> S_AXIS_din_tuser/1
  S_AXIS_din_tlast_/1 -> S_AXIS_din_tlast/1
  Constant3/1 -> S_AXIS_enable/1
  Constant2/1 -> S_AXIS_aresetn/1
  Constant1/1 -> M_AXIS_dout_tready/1
  Constant/1 -> S_AXIS_din_tvalid/1
  Vitis HLS Input/1 -> Versal RF FFT/1(dout_tready)
  Vitis HLS Input/3 -> Versal RF FFT/2(aresetn)
  Vitis HLS Input/5 -> Versal RF FFT/3(tdata_imag_3)
  Vitis HLS Input/7 -> Versal RF FFT/4(tdata_real_3)
  Vitis HLS Input/9 -> Versal RF FFT/5(tdata_imag_2)
  Vitis HLS Input/11 -> Versal RF FFT/6(tdata_real_2)
  Vitis HLS Input/13 -> Versal RF FFT/7(tdata_imag_1)
  Vitis HLS Input/15 -> Versal RF FFT/8(tdata_real_1)
  Vitis HLS Input/17 -> Versal RF FFT/9(tdata_imag_0)
  Vitis HLS Input/19 -> Versal RF FFT/10(tdata_real_0)
  Vitis HLS Input/21 -> Versal RF FFT/11(din_tlast)
  Vitis HLS Input/23 -> Versal RF FFT/12(tuser_scaling)
  Vitis HLS Input/25 -> Versal RF FFT/13(tuser_direction)
  Vitis HLS Input/27 -> Versal RF FFT/14(tuser_point_size)
  Vitis HLS Input/29 -> Versal RF FFT/15(din_tvalid)
  Vitis HLS Input/31 -> Versal RF FFT/16(din_enable)
  Vitis HLS Input/2 -> Terminator4/1
  Vitis HLS Input/4 -> Terminator5/1
  Vitis HLS Input/6 -> Terminator6/1
  Vitis HLS Input/8 -> Terminator7/1
  Vitis HLS Input/10 -> Terminator8/1
  Vitis HLS Input/12 -> Terminator9/1
  Vitis HLS Input/14 -> Terminator10/1
  Vitis HLS Input/16 -> Terminator11/1
  Vitis HLS Input/18 -> Terminator12/1
  Vitis HLS Input/20 -> Terminator13/1
  Vitis HLS Input/22 -> Terminator14/1
  Vitis HLS Input/24 -> Terminator15/1
  Vitis HLS Input/26 -> Terminator16/1
  Vitis HLS Input/28 -> Terminator17/1
  Vitis HLS Input/30 -> Terminator18/1
  Vitis HLS Input/32 -> Terminator19/1
  Versal RF FFT/17(din_tready) -> Vitis HLS Output/17
  Versal RF FFT/16(dout_tvalid) -> Vitis HLS Output/16
  Versal RF FFT/15(dout_tuser_point_size) -> Vitis HLS Output/15
  Versal RF FFT/14(dout_tuser_direction) -> Vitis HLS Output/14
  Versal RF FFT/13(tuser_index_0) -> Vitis HLS Output/13
  Versal RF FFT/12(tuser_index_1) -> Vitis HLS Output/12
  Versal RF FFT/11(tuser_index_2) -> Vitis HLS Output/11
  Versal RF FFT/10(tuser_index_3) -> Vitis HLS Output/10
  Versal RF FFT/9(dout_tlast) -> Vitis HLS Output/9
  Versal RF FFT/1(imag_3) -> Vitis HLS Output/1
  Versal RF FFT/2(real_3) -> Vitis HLS Output/2
  Versal RF FFT/3(imag_2) -> Vitis HLS Output/3
  Versal RF FFT/4(real_2) -> Vitis HLS Output/4
  Versal RF FFT/5(imag_1) -> Vitis HLS Output/5
  Versal RF FFT/6(real_1) -> Vitis HLS Output/6
  Versal RF FFT/7(imag_0) -> Vitis HLS Output/7
  Versal RF FFT/8(real_0) -> Vitis HLS Output/8
  Vitis HLS Output/2 -> Terminator20/1
  S_AXIS_din_tdata/1 -> Shift/1
  S_AXIS_enable/1 -> Vitis HLS Input/7
  S_AXIS_aresetn/1 -> Vitis HLS Input/6
  S_AXIS_din_tlast/1 -> Vitis HLS Input/5
  S_AXIS_din_tuser/1 -> Vitis HLS Input/4
  S_AXIS_din_tvalid/1 -> Vitis HLS Input/3
  M_AXIS_dout_tready/1 -> Vitis HLS Input/2
  Vitis HLS Output/3 -> M_AXIS_dout_tlast/1
  Vitis HLS Output/9 -> M_AXIS_dout_tvalid/1
  Vitis HLS Output/7 -> M_AXIS_dout_tuser/1
  M_AXIS_dout_tlast/1 -> Scope1/1
  Vitis HLS Output/5 -> S_AXIS_din_tready/1
  M_AXIS_dout_tuser/1 -> Scope1/3
  M_AXIS_dout_tvalid/1 -> tvalid/1, Scope1/4
  Constant4/1 -> Vitis HLS Input/8
  Constant5/1 -> Vitis HLS Output/18
  S_AXIS_din_tready/1 -> Scope1/2
  Shift/1 -> Vitis HLS Input/1
  Data Type Conversion/1 -> Abs/1

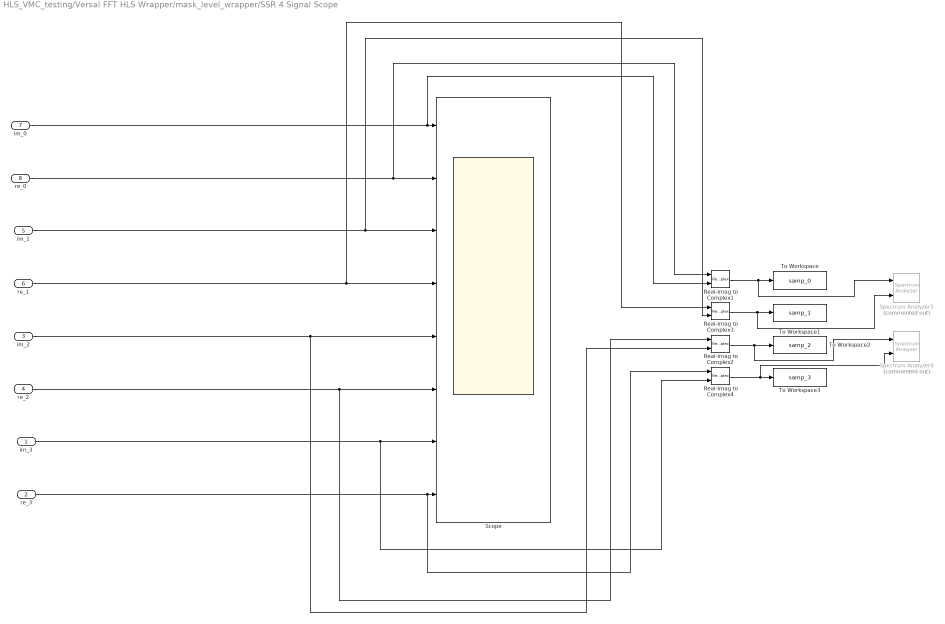
== system HLS_VMC_testing/Versal FFT HLS Wrapper/mask_level_wrapper/SSR 4 Signal Scope ==
  im_3 : Inport
  re_3 : Inport  Port=2
  im_2 : Inport  Port=3
  re_2 : Inport  Port=4
  im_1 : Inport  Port=5
  re_1 : Inport  Port=6
  im_0 : Inport  Port=7
  re_0 : Inport  Port=8
  Real-Imag to Complex{1..4} (4 alike) : RealImagToComplex
  Scope : Scope  NumInputPorts=8
      settings: ActiveDisplayYMinimum=-1.2499961853027344  ActiveDisplayYMaximum=1.2499656677246094
  Spectrum Analyzer4 : SpectrumAnalyzer  Commented=on  NumInputPorts=2  WindowPosition=[1.000000,1.000000,2560.000000,1389.000000,]  ScopeFrameLocation=window  ViewType=Spectrum and spectrogram  WindowInvariantSamplesPerUpdate=on  YLimits=[-3606.821 430.7673]  ColorLimits=[-3606.821 430.7673]
  Spectrum Analyzer5 : SpectrumAnalyzer  Commented=on  NumInputPorts=2  WindowPosition=[1.000000,1.000000,2560.000000,1389.000000,]  ScopeFrameLocation=window  ViewType=Spectrum and spectrogram  WindowInvariantSamplesPerUpdate=on  YLimits=[-3606.5845 428.6394]  ColorLimits=[-3606.5845 428.6394]
  To Workspace : ToWorkspace  VariableName=samp_0  SaveFormat=Structure With Time  SampleTime=-1
  To Workspace1 : ToWorkspace  VariableName=samp_1  SaveFormat=Structure With Time  SampleTime=-1
  To Workspace2 : ToWorkspace  VariableName=samp_2  SaveFormat=Structure With Time  SampleTime=-1
  To Workspace3 : ToWorkspace  VariableName=samp_3  SaveFormat=Structure With Time  SampleTime=-1
  wires:
  Real-Imag to Complex3/1 -> Spectrum Analyzer5/2, To Workspace1/1
  Real-Imag to Complex1/1 -> Spectrum Analyzer5/1, To Workspace/1
  re_3/1 -> Real-Imag to Complex4/1, Scope/8
  Real-Imag to Complex4/1 -> Spectrum Analyzer4/2, To Workspace3/1
  re_2/1 -> Real-Imag to Complex2/1, Scope/6
  im_2/1 -> Real-Imag to Complex2/2, Scope/5
  re_0/1 -> Real-Imag to Complex1/1, Scope/2
  im_3/1 -> Real-Imag to Complex4/2, Scope/7
  Real-Imag to Complex2/1 -> Spectrum Analyzer4/1, To Workspace2/1
  im_1/1 -> Real-Imag to Complex3/2, Scope/3
  re_1/1 -> Real-Imag to Complex3/1, Scope/4
  im_0/1 -> Real-Imag to Complex1/2, Scope/1

== system HLS_VMC_testing/Versal FFT HLS Wrapper/mask_level_wrapper/Subsystem ==
  In1 : Inport
  In2 : Inport  Port=2
  In3 : Inport  Port=3
  In4 : Inport  Port=4
  In5 : Inport  Port=5
  In6 : Inport  Port=6
  In7 : Inport  Port=7
  In8 : Inport  Port=8
  Display{,1..7} (8 alike) : Display
  wires:
  In1/1 -> Display/1
  In2/1 -> Display1/1
  In8/1 -> Display7/1
  In6/1 -> Display5/1
  In7/1 -> Display6/1
  In5/1 -> Display4/1
  In4/1 -> Display3/1
  In3/1 -> Display2/1
